simulink model "skipper_lqr_2"  (R2024b)
settings: Solver=FixedStepAuto  StartTime=0.0  StopTime=20  RelTol=1e-3
values from neighbouring files (symbols this model uses):
  A = zeros(12, 12)    [eomStateSpace.m]    (also in lqrMatrices.m = [)
  B = zeros(12, 5)    [eomStateSpace.m]    (also in lqrMatrices.m = [)
  C = diag(ones(1, 12))    [eomStateSpace.m]    (also in lqrMatrices.m)
  d = [ ... (first row only)    [lqrMatrices.m]
  D = zeros(size(B))    [eomStateSpace.m]    (also in lqrMatrices.m)
  g = constants(2)    [eomSims.m]
  K = lqr(sys, Q, R)    [eomStateSpace.m]    (also in lqrMatrices.m)
  M = constants(1)    [eomSims.m]
undefined symbols (not defined in the file or in its folder): Uff
settings Model: Creator=nehir  LastModifiedBy=nehir
settings OptimizationCC: OptimizeBlockIOStorage=off  OptimizeDataStoreBuffers=off  BusAssignmentInplaceUpdate=off
settings DebuggingCC: SFUnexpectedBacktrackingDiag=warning  SFNoUnconditionalDefaultTransitionDiag=warning
settings RTWCC: GenerateReport=on  BuildConfiguration=Debug  LaunchReport=on
settings CodeAppCC: ForceParamTrailComments=on  MATLABSourceComments=on  EnableCustomComments=on
settings GRTTargetCC: CombineSignalStateStructs=on  SupportVariableSizeSignals=on  MultiInstanceErrorCode=Warning

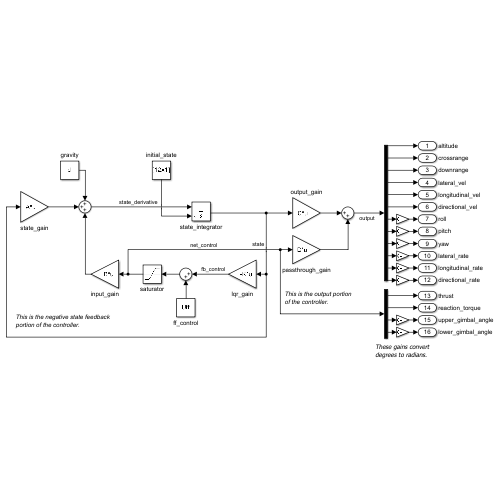
[thumbnail: Simulink's stored preview of the top-level diagram]
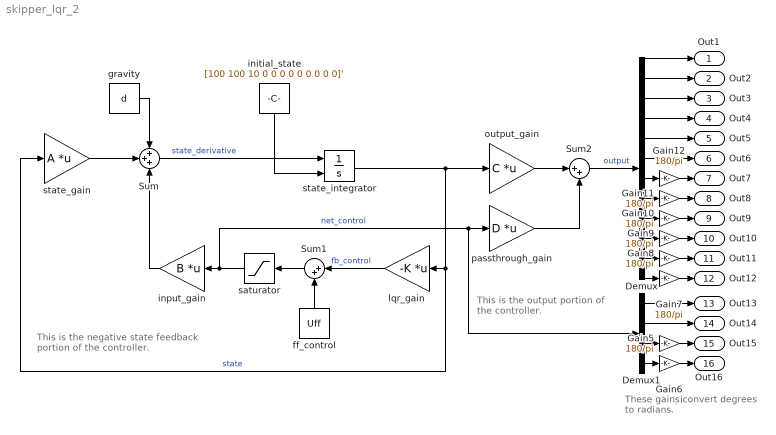
== system skipper_lqr_2 ==
  note: This is the negative state feedback
      | portion of the controller.
  note: These gains convert
      | degrees to radians.
  note: This is the output portion
      | of the controller.
  Demux : Demux  Outputs=12
  Demux1 : Demux
  Gain{5..12} (8 alike) : Gain  Gain=180/pi
  Sum : Sum  Inputs=+++
  Sum1 : Sum  Inputs=|++
  Sum2 : Sum  Inputs=|++
  ff_control : Constant  Value=Uff
  gravity : Constant  Value=d  OutDataTypeStr=double
  initial_state : Constant  Value=[100 100 10 0 0 0 0 0 0 0 0 0]'
  input_gain : Gain  Gain=B  Multiplication=Matrix(K*u)
  lqr_gain : Gain  Gain=-K  Multiplication=Matrix(K*u)
  output_gain : Gain  Gain=C  Multiplication=Matrix(K*u)
  passthrough_gain : Gain  Gain=D  Multiplication=Matrix(K*u)
  saturator : Saturate  UpperLimit=[M*g*4 1 pi/22 pi/22]  LowerLimit=[0 -1 -pi/22 -pi/22]
  state_gain : Gain  Gain=A  Multiplication=Matrix(K*u)
  state_integrator : Integrator  InitialConditionSource=external  InitialCondition=zeros(12, 1)
  Out1 : Outport  SignalName=altitude  Unit=ft
  Out2 : Outport  Port=2  SignalName=crossrange  Unit=ft
  Out3 : Outport  Port=3  SignalName=downrange  Unit=ft
  Out4 : Outport  Port=4  SignalName=lateral_vel  Unit=ft/s
  Out5 : Outport  Port=5  SignalName=longitudinal_vel  Unit=ft/s
  Out6 : Outport  Port=6  SignalName=directional_vel  Unit=ft/s
  Out7 : Outport  Port=7  SignalName=roll  Unit=deg
  Out8 : Outport  Port=8  SignalName=pitch  Unit=deg
  Out9 : Outport  Port=9  SignalName=yaw  Unit=deg
  Out10 : Outport  Port=10  SignalName=lateral_rate  Unit=deg/s
  Out11 : Outport  Port=11  SignalName=longitudinal_rate  Unit=deg/s
  Out12 : Outport  Port=12  SignalName=directional_rate  Unit=deg/s
  Out13 : Outport  Port=13  SignalName=thrust  Unit=lbf
  Out14 : Outport  Port=14  SignalName=reaction_torque  Unit=lbf*ft
  Out15 : Outport  Port=15  SignalName=upper_gimbal_angle  Unit=deg
  Out16 : Outport  Port=16  SignalName=lower_gimbal_angle  Unit=deg
  wires:
  Demux1/2 -> Out14/1
  Gain6/1 -> Out16/1
  Sum2/1 -> Demux/1  "output"
  Demux/3 -> Out3/1
  ff_control/1 -> Sum1/2
  Demux/12 -> Gain7/1
  Demux/10 -> Gain9/1
  passthrough_gain/1 -> Sum2/2
  Demux/7 -> Gain12/1
  input_gain/1 -> Sum/3
  Gain5/1 -> Out15/1
  initial_state/1 -> state_integrator/2
  Sum/1 -> state_integrator/1  "state_derivative"
  Demux/4 -> Out4/1
  Demux/9 -> Gain10/1
  lqr_gain/1 -> Sum1/1  "fb_control"
  Gain11/1 -> Out8/1
  Demux/1 -> Out1/1
  state_integrator/1 -> lqr_gain/1, state_gain/1, output_gain/1  "state"
  saturator/1 -> Demux1/1, passthrough_gain/1, input_gain/1  "net_control"
  Demux1/3 -> Gain5/1
  Demux/8 -> Gain11/1
  Demux1/4 -> Gain6/1
  Demux1/1 -> Out13/1
  Demux/5 -> Out5/1
  Gain9/1 -> Out10/1
  Demux/6 -> Out6/1
  Gain10/1 -> Out9/1
  output_gain/1 -> Sum2/1
  state_gain/1 -> Sum/2
  Demux/11 -> Gain8/1
  Sum1/1 -> saturator/1
  Gain8/1 -> Out11/1
  Gain7/1 -> Out12/1
  gravity/1 -> Sum/1
  Demux/2 -> Out2/1
  Gain12/1 -> Out7/1
